simulink model "circleControlLoop"  (Simulink 7.5)
settings: Solver=ode1  StartTime=0.0  StopTime=15  FixedStep=0.001  RelTol=1e-3
PostLoadFcn:
  | , if any(exist('dsrtsu_mdlpostloadfcn', 'file') == [2, 3, 6]), try dsrtsu_mdlpostloadfcn('Execute', bdroot); catch fprintf('Error in PostLoadFcn (dsrtsu_mdlpostloadfcn) for model "%s":\n %s\n', bdroot, lasterr); end, end,
values from neighbouring files (symbols this model uses):
  kn = 1    [main.m]
  kt = 10    [main.m]
  r0 = Re-3.5    [main.m]
  Ts = 0.001    [main.m]
  Xr = [circXt.',circYt.',circXtd,circYtd,circXtdd,circYtdd]    [getCircle.m]
undefined symbols (not defined in the file or in its folder): DiscIntNeverNeededParam, xc, yc
libraries: rtilib1103 x12
settings Model: DSRTSU_INTERNAL_RTI_VER=360  DSRTSU_INTERNAL_RTI_TYPE=rti1103  Creator=daq  LastModifiedBy=daq  BufferReuse=off
settings OptimizationCC: BlockReduction=off  OptimizeBlockIOStorage=off  BufferReuse=off  ExpressionFolding=off  LocalBlockOutputs=off
settings HardwareCC: ProdIntDivRoundTo=Zero  ProdEndianess=BigEndian  ProdHWDeviceType=Generic->Custom  TargetIntDivRoundTo=Zero  TargetEndianess=BigEndian  TargetHWDeviceType=Generic->Custom
settings RTWCC: SystemTargetFile=rti1103.tlc  MakeCommand=make_rti  TemplateMakefile=rti1103.tmf  Description=dSPACE DS1103 Hardware Platform  ProcessScript=rti1103_make_rtw_hook
settings STFCustomTargetCC: ParMdlRefBuildCompliant=on  GeneratePreprocessorConditionals=Disable all  MatFileLogging=on  SystemTargetFile=rti1103.tlc
settings GRTTargetCC: CompOptLevelCompliant=off  ExtModeMexFile=noextcomm
settings CustomProperty: DataType=RTWOptions_EnumType_C__dSPACE_matlab_rti1103_tlc_rti1103_1InitialSimState  Value=RUN
settings EnumStrPairs: String=RUN

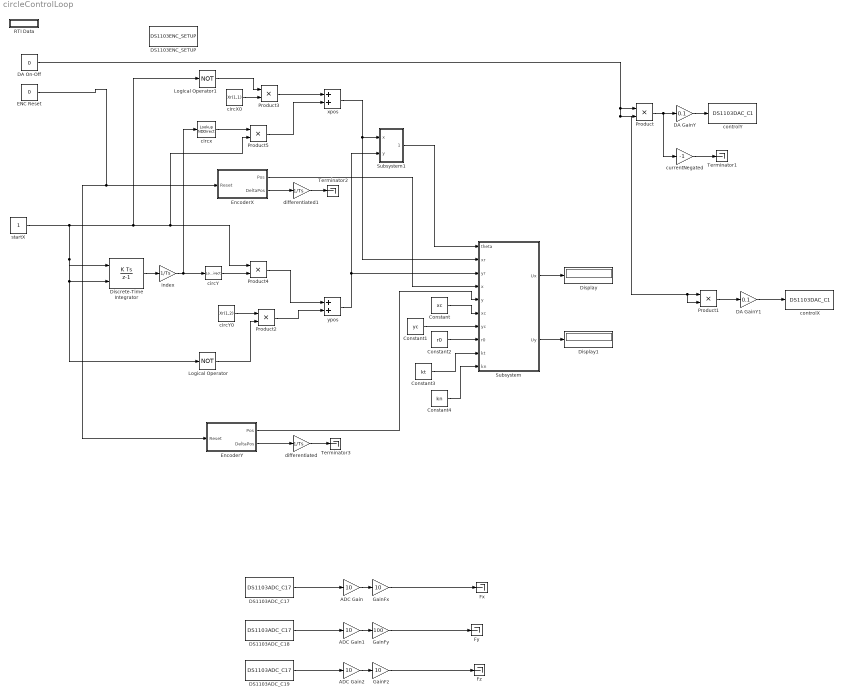
== system circleControlLoop ==
  " EncoderX" : Subsystem
  " EncoderY" : Subsystem
  ADC Gain : Gain  Gain=10  ParameterDataType=fixdt(1, 16)  ParameterScaling=2^0  OutDataType=fixdt(1, 16)  OutScaling=2^0
  ADC Gain1 : Gain  Gain=10  ParameterDataType=fixdt(1, 16)  ParameterScaling=2^0  OutDataType=fixdt(1, 16)  OutScaling=2^0
  ADC Gain2 : Gain  Gain=10  ParameterDataType=fixdt(1, 16)  ParameterScaling=2^0  OutDataType=fixdt(1, 16)  OutScaling=2^0
  Constant : Constant  Value=xc  OutDataType=fixdt(1, 16)  OutScaling=2^0
  Constant1 : Constant  Value=yc  OutDataType=fixdt(1, 16)  OutScaling=2^0
  Constant2 : Constant  Value=r0  OutDataType=fixdt(1, 16)  OutScaling=2^0
  Constant3 : Constant  Value=kt  OutDataType=fixdt(1, 16)  OutScaling=2^0
  Constant4 : Constant  Value=kn  OutDataType=fixdt(1, 16)  OutScaling=2^0
  DA GainY : Gain  Gain=0.1  ParameterDataType=fixdt(1, 16)  ParameterScaling=2^0  OutDataType=fixdt(1, 16)  OutScaling=2^0
  DA GainY1 : Gain  Gain=0.1  ParameterDataType=fixdt(1, 16)  ParameterScaling=2^0  OutDataType=fixdt(1, 16)  OutScaling=2^0
  DA On-Off : Constant  Value=0  OutDataType=fixdt(1, 16)  OutScaling=2^0
  DS1103ADC_C17 : rtilib1103/DS1103 MASTER PPC/DS1103ADC_C17  SystemSampleTime=-1  ChannelNo=17  TimerAPreTrigger=0  Reserved2=[]  Reserved3=[]  Reserved4=[]  DialogFcn=gui1103adc  UnitName={ 'DS1103ADC_C' }  UnitValues={ 17 }  DSProperties=struct('RTI',struct('Version',uint32(1),'BlockType',struct('isSLSource',uint8(1),'isSLSink',uint8(0),'isHWSource',uint8(1),'isHWSink',uint8(0),'isSetup',uint8(0),'isInline',uint8(1),'isNonInline',uint8(0),'isInterrupt',uint8(0),'isChannelwise',uint8(1)),'IOBoardType','DS1103MASTER','UnitType','ADC','Identifier','ADC','DialogType','ML','BlockSet','NONE','SlaveProcessor','NONE'))
  DS1103ADC_C18 : rtilib1103/DS1103 MASTER PPC/DS1103ADC_C17  SystemSampleTime=-1  ChannelNo=18  TimerAPreTrigger=0  Reserved2=[]  Reserved3=[]  Reserved4=[]  DialogFcn=gui1103adc  UnitName={ 'DS1103ADC_C' }  UnitValues={ 18 }  DSProperties=struct('RTI',struct('Version',uint32(1),'BlockType',struct('isSLSource',uint8(1),'isSLSink',uint8(0),'isHWSource',uint8(1),'isHWSink',uint8(0),'isSetup',uint8(0),'isInline',uint8(1),'isNonInline',uint8(0),'isInterrupt',uint8(0),'isChannelwise',uint8(1)),'IOBoardType','DS1103MASTER','UnitType','ADC','Identifier','ADC','DialogType','ML','BlockSet','NONE','SlaveProcessor','NONE'))
  DS1103ADC_C19 : rtilib1103/DS1103 MASTER PPC/DS1103ADC_C17  SystemSampleTime=-1  ChannelNo=19  TimerAPreTrigger=0  Reserved2=[]  Reserved3=[]  Reserved4=[]  DialogFcn=gui1103adc  UnitName={ 'DS1103ADC_C' }  UnitValues={ 19 }  DSProperties=struct('RTI',struct('Version',uint32(1),'BlockType',struct('isSLSource',uint8(1),'isSLSink',uint8(0),'isHWSource',uint8(1),'isHWSink',uint8(0),'isSetup',uint8(0),'isInline',uint8(1),'isNonInline',uint8(0),'isInterrupt',uint8(0),'isChannelwise',uint8(1)),'IOBoardType','DS1103MASTER','UnitType','ADC','Identifier','ADC','DialogType','ML','BlockSet','NONE','SlaveProcessor','NONE'))
  DS1103ENC_SETUP : rtilib1103/DS1103 MASTER PPC/DS1103ENC_SETUP  SystemSampleTime=-1  EncRange=0  Reserved1=[]  Reserved2=[]  Reserved3=[]  Reserved4=[]  DialogFcn=gui1103enc_setup  UnitName={ 'DS1103ENC_SETUP' }  UnitValues={ [] }  DSProperties=struct('RTI',struct('Version',uint32(1),'BlockType',struct('isSLSource',uint8(0),'isSLSink',uint8(0),'isHWSource',uint8(0),'isHWSink',uint8(0),'isSetup',uint8(0),'isInline',uint8(1),'isNonInline',uint8(0),'isInterrupt',uint8(0),'isChannelwise',uint8(0)),'IOBoardType','DS1103MASTER','UnitType','ENC','Identifier','ENCMASTER','DialogType','ML','BlockSet','NONE','SlaveProcessor','NONE'))
      settings: SignalType=[0 0 0 0 0 0 0]
  Discrete-Time Integrator : DiscreteIntegrator  ExternalReset=rising  SampleTime=Ts  OutDataType=fixdt(1, 16)  OutScaling=2^0  ICPrevOutput=DiscIntNeverNeededParam  ICPrevScaledInput=DiscIntNeverNeededParam
  Display : Display
  Display1 : Display
  ENC Reset : Constant  Value=0  OutDataType=fixdt(1, 16)  OutScaling=2^0
  Fx : Terminator
  Fy : Terminator
  Fz : Terminator
  GainFx : Gain  Gain=10  ParameterDataType=fixdt(1, 16)  ParameterScaling=2^0  OutDataType=fixdt(1, 16)  OutScaling=2^0
  GainFy : Gain  Gain=100  ParameterDataType=fixdt(1, 16)  ParameterScaling=2^0  OutDataType=fixdt(1, 16)  OutScaling=2^0
  GainFz : Gain  Gain=10  ParameterDataType=fixdt(1, 16)  ParameterScaling=2^0  OutDataType=fixdt(1, 16)  OutScaling=2^0
  Logical Operator : Logic  Operator=NOT  AllPortsSameDT=off  OutDataTypeMode=boolean  LogicDataType=fixdt(0, 8)  OutDataTypeStr=boolean
  Logical Operator1 : Logic  Operator=NOT  AllPortsSameDT=off  OutDataTypeMode=boolean  LogicDataType=fixdt(0, 8)  OutDataTypeStr=boolean
  Product{,1..5} (6 alike) : Product  OutDataType=fixdt(1, 16)  OutScaling=2^0  RndMeth=Zero
  RTI Data : Subsystem  Tag=struct('RTIDataServer',struct('RTIDataServerVs','2','RTIModelDescription','struct(''main'',''circleControlLoop'',''sub'',''circleControlLoop'',''isMp'',0)'))  LoadFcn="if exist('rtidc'), try,  rtidc('DataHostBlockClbLoad', gcbh); catch, disp(['Warning: ''LoadFcn'' for RTI Data block failed: ' lasterr]); end, end,"
      settings: CopyFcn="if exist('rtidc'), try,  rtidc('DataHostBlockClbCopy', gcbh); catch, disp(['Warning: ''CopyFcn'' for RTI Data block failed: ' lasterr]); end, end,"  DeleteFcn="if exist('rtidc'), try,  rtidc('DataHostBlockClbDelete', gcbh); catch, disp(['Warning: ''DeleteFcn'' for RTI Data block failed: ' lasterr]); end, end,"  ModelCloseFcn="if exist('rtidc'), try,  rtidc('DataHostBlockClbModelClose', gcbh); catch, disp(['Warning: ''ModelCloseFcn'' for RTI Data block failed: ' lasterr]); end, end,"  PreSaveFcn="if exist('rtidc'), try,  rtidc('DataHostBlockClbPreSave', gcbh); catch, disp(['Warning: ''PreSaveFcn'' for RTI Data block failed: ' lasterr]); end, end,"  PostSaveFcn="if exist('rtidc'), try,  rtidc('DataHostBlockClbPostSave', gcbh); catch, disp(['Warning: ''PostSaveFcn'' for RTI Data block failed: ' lasterr]); end, end,"  NameChangeFcn="if exist('rtidc'), try,  rtidc('DataHostBlockClbNameChange', gcbh); catch, disp(['Warning: ''NameChangeFcn'' for RTI Data block failed: ' lasterr]); end, end,"
      mask Type: RTI_DATA_HOST
      mask Description:
      | RTI Data Block.
      | This block is used by RTI to store internal model-dependent data.
      | Please keep this block on the root level of the model. Deleting this block will result in data loss.
      | 
      | NEVER DELETE OR COPY THIS BLOCK!
      mask Help:
      | RTI Data Block.
      | This block is used by RTI to store internal model-dependent data.
      | Please keep this block on the root level of the model. Deleting this block will result in data loss.
      | 
      | NEVER DELETE OR COPY THIS BLOCK!
      mask Display:
      | text(0.5, 0.5, 'RTI Data', 'HorizontalAlignment', 'center');
      | plot([1 0]);
  Subsystem : Subsystem
  Subsystem1 : Subsystem
  Terminator1 : Terminator
  Terminator2 : Terminator
  Terminator3 : Terminator
  circX0 : Constant  Value=Xr(1,1)  OutDataType=fixdt(1, 16)  OutScaling=2^0
  circY : LookupNDDirect  NumberOfTableDimensions=1  Table=Xr(:,2)
  circY0 : Constant  Value=Xr(1,2)  OutDataType=fixdt(1, 16)  OutScaling=2^0
  circx : LookupNDDirect  NumberOfTableDimensions=1  Table=Xr(:,1)
  controlX : rtilib1103/DS1103 MASTER PPC/DS1103DAC_C1  SystemSampleTime=-1  ChannelNo=1  InitValue=0  TermMode=0  TermValue=0  Reserved1=[]  Reserved2=[]  Reserved3=[]  Reserved4=[]  DialogFcn=gui1103dac  UnitName={ 'DS1103DAC_C' }  UnitValues={ 1 }  DSProperties=struct('RTI',struct('Version',uint32(1),'BlockType',struct('isSLSource',uint8(0),'isSLSink',uint8(1),'isHWSource',uint8(0),'isHWSink',uint8(1),'isSetup',uint8(0),'isInline',uint8(1),'isNonInline',uint8(0),'isInterrupt',uint8(0),'isChannelwise',uint8(1)),'IOBoardType','DS1103MASTER','UnitType','DAC','Identifier','DAC','DialogType','ML','BlockSet','NONE','SlaveProcessor','NONE'))
  controlY : rtilib1103/DS1103 MASTER PPC/DS1103DAC_C1  SystemSampleTime=-1  ChannelNo=2  InitValue=0  TermMode=1  TermValue=0  Reserved1=[]  Reserved2=[]  Reserved3=[]  Reserved4=[]  DialogFcn=gui1103dac  UnitName={ 'DS1103DAC_C' }  UnitValues={ 2 }  DSProperties=struct('RTI',struct('Version',uint32(1),'BlockType',struct('isSLSource',uint8(0),'isSLSink',uint8(1),'isHWSource',uint8(0),'isHWSink',uint8(1),'isSetup',uint8(0),'isInline',uint8(1),'isNonInline',uint8(0),'isInterrupt',uint8(0),'isChannelwise',uint8(1)),'IOBoardType','DS1103MASTER','UnitType','DAC','Identifier','DAC','DialogType','ML','BlockSet','NONE','SlaveProcessor','NONE'))
  currentNegated : Gain  Gain=-1  ParameterDataType=fixdt(1, 16)  ParameterScaling=2^0  OutDataType=fixdt(1, 16)  OutScaling=2^0
  differentiated : Gain  Gain=1/Ts  ParameterDataType=fixdt(1, 16)  ParameterScaling=2^0  OutDataType=fixdt(1, 16)  OutScaling=2^0
  differentiated1 : Gain  Gain=1/Ts  ParameterDataType=fixdt(1, 16)  ParameterScaling=2^0  OutDataType=fixdt(1, 16)  OutScaling=2^0
  index : Gain  Gain=1/Ts  ParameterDataType=fixdt(1, 16)  ParameterScaling=2^0  OutDataType=fixdt(1, 16)  OutScaling=2^0
  startX : Constant  OutDataType=fixdt(1, 16)  OutScaling=2^0
  xpos : Sum  OutDataType=fixdt(1, 16)  OutScaling=2^-10
  ypos : Sum  OutDataType=fixdt(1, 16)  OutScaling=2^-10
  wires:
  DA GainY/1 -> controlY/1
  Product/1 -> DA GainY/1, currentNegated/1
  DA On-Off/1 -> Product/1, Product/2, Product1/1, Product1/2
  ENC Reset/1 -> " EncoderX"/1(Reset), " EncoderY"/1(Reset)
  DS1103ADC_C18/1 -> ADC Gain1/1
  GainFz/1 -> Fz/1
  DS1103ADC_C17/1 -> ADC Gain/1
  ADC Gain/1 -> GainFx/1
  ADC Gain1/1 -> GainFy/1
  ADC Gain2/1 -> GainFz/1
  GainFy/1 -> Fy/1
  currentNegated/1 -> Terminator1/1
  " EncoderY"/2(DeltaPos) -> differentiated/1
  GainFx/1 -> Fx/1
  DS1103ADC_C19/1 -> ADC Gain2/1
  startX/1 -> Discrete-Time Integrator/1, Discrete-Time Integrator/2, Logical Operator/1, Logical Operator1/1, Product4/1, Product5/2
  Discrete-Time Integrator/1 -> index/1
  index/1 -> circY/1, circx/1
  differentiated1/1 -> Terminator2/1
  differentiated/1 -> Terminator3/1
  Product1/1 -> DA GainY1/1
  DA GainY1/1 -> controlX/1
  circY0/1 -> Product2/1
  Product2/1 -> ypos/2
  Logical Operator/1 -> Product2/2
  circX0/1 -> Product3/2
  Product3/1 -> xpos/1
  Logical Operator1/1 -> Product3/1
  circY/1 -> Product4/2
  Product4/1 -> ypos/1
  circx/1 -> Product5/1
  Product5/1 -> xpos/2
  " EncoderX"/2(DeltaPos) -> differentiated1/1
  xpos/1 -> Subsystem/2(xr), Subsystem1/1(x)
  ypos/1 -> Subsystem1/2(y), Subsystem/3(yr)
  Subsystem1/1(Out1) -> Subsystem/1(theta)
  " EncoderX"/1(Pos) -> Subsystem/4(x)
  " EncoderY"/1(Pos) -> Subsystem/5(y)
  Constant/1 -> Subsystem/6(xc)
  Constant1/1 -> Subsystem/7(yc)
  Constant2/1 -> Subsystem/8(r0)
  Constant3/1 -> Subsystem/9(kt)
  Constant4/1 -> Subsystem/10(kn)
  Subsystem/1(Ux) -> Display/1
  Subsystem/2(Uy) -> Display1/1

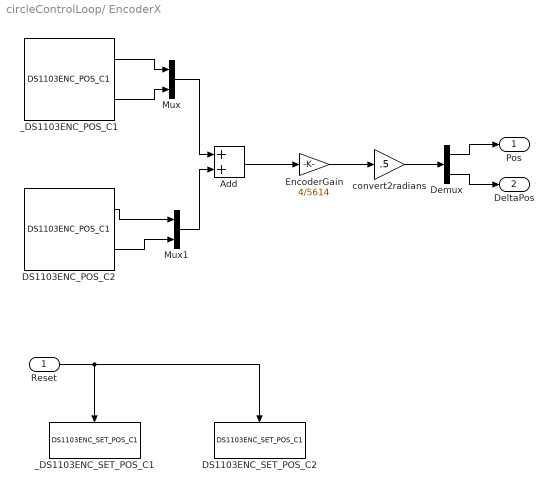
== system circleControlLoop/ EncoderX ==
  Reset : Inport
  Add : Sum  OutDataType=fixdt(1, 16)  OutScaling=2^-10
  DS1103ENC_POS_C2 : rtilib1103/DS1103 MASTER PPC/DS1103ENC_POS_C1  SystemSampleTime=-1  ChannelNo=2  PosValue=0  Reserved1=[]  Reserved2=[]  Reserved3=[]  Reserved4=[]  DialogFcn=gui1103enc_pos  UnitName={ 'DS1103ENC_POS_C' }  UnitValues={ 2 }  DSProperties=struct('RTI',struct('Version',uint32(1),'BlockType',struct('isSLSource',uint8(1),'isSLSink',uint8(0),'isHWSource',uint8(1),'isHWSink',uint8(0),'isSetup',uint8(0),'isInline',uint8(1),'isNonInline',uint8(0),'isInterrupt',uint8(0),'isChannelwise',uint8(1)),'IOBoardType','DS1103MASTER','UnitType','ENC','Identifier','ENCPOSCH','DialogType','ML','BlockSet','NONE','SlaveProcessor','NONE'))
  DS1103ENC_SET_POS_C2 : rtilib1103/DS1103 MASTER PPC/DS1103ENC_SET_POS_C1  SystemSampleTime=-1  ChannelNo=2  PosValue=0  Reserved1=[]  Reserved2=[]  Reserved3=[]  Reserved4=[]  DialogFcn=gui1103enc_set_pos  UnitName={ 'DS1103ENC_SET_POS_C' }  UnitValues={ 2 }  DSProperties=struct('RTI',struct('Version',uint32(1),'BlockType',struct('isSLSource',uint8(0),'isSLSink',uint8(1),'isHWSource',uint8(0),'isHWSink',uint8(1),'isSetup',uint8(0),'isInline',uint8(1),'isNonInline',uint8(0),'isInterrupt',uint8(0),'isChannelwise',uint8(1)),'IOBoardType','DS1103MASTER','UnitType','ENC','Identifier','ENCRESET','DialogType','ML','BlockSet','NONE','SlaveProcessor','NONE'))
  Demux : Demux  Outputs=2
  EncoderGain : Gain  Gain=4/5614  SaturateOnIntegerOverflow=on  OutDataTypeStr=Inherit: Same as input  ParamDataTypeStr=Inherit: Same as input
  Mux : Mux  Inputs=2
  Mux1 : Mux  Inputs=2
  _DS1103ENC_POS_C1 : rtilib1103/DS1103 MASTER PPC/DS1103ENC_POS_C1  SystemSampleTime=-1  ChannelNo=1  PosValue=0  Reserved1=[]  Reserved2=[]  Reserved3=[]  Reserved4=[]  DialogFcn=gui1103enc_pos  UnitName={ 'DS1103ENC_POS_C' }  UnitValues={ 1 }  DSProperties=struct('RTI',struct('Version',uint32(1),'BlockType',struct('isSLSource',uint8(1),'isSLSink',uint8(0),'isHWSource',uint8(1),'isHWSink',uint8(0),'isSetup',uint8(0),'isInline',uint8(1),'isNonInline',uint8(0),'isInterrupt',uint8(0),'isChannelwise',uint8(1)),'IOBoardType','DS1103MASTER','UnitType','ENC','Identifier','ENCPOSCH','DialogType','ML','BlockSet','NONE','SlaveProcessor','NONE'))
  _DS1103ENC_SET_POS_C1 : rtilib1103/DS1103 MASTER PPC/DS1103ENC_SET_POS_C1  SystemSampleTime=-1  ChannelNo=1  PosValue=0  Reserved1=[]  Reserved2=[]  Reserved3=[]  Reserved4=[]  DialogFcn=gui1103enc_set_pos  UnitName={ 'DS1103ENC_SET_POS_C' }  UnitValues={ 1 }  DSProperties=struct('RTI',struct('Version',uint32(1),'BlockType',struct('isSLSource',uint8(0),'isSLSink',uint8(1),'isHWSource',uint8(0),'isHWSink',uint8(1),'isSetup',uint8(0),'isInline',uint8(1),'isNonInline',uint8(0),'isInterrupt',uint8(0),'isChannelwise',uint8(1)),'IOBoardType','DS1103MASTER','UnitType','ENC','Identifier','ENCRESET','DialogType','ML','BlockSet','NONE','SlaveProcessor','NONE'))
  "convert2radians " : Gain  Gain=.5
  Pos : Outport
  DeltaPos : Outport  Port=2
  wires:
  _DS1103ENC_POS_C1/1 -> Mux/1
  _DS1103ENC_POS_C1/2 -> Mux/2
  EncoderGain/1 -> "convert2radians "/1
  "convert2radians "/1 -> Demux/1
  Reset/1 -> _DS1103ENC_SET_POS_C1/Trigger, DS1103ENC_SET_POS_C2/Trigger
  Mux/1 -> Add/1
  Demux/1 -> Pos/1
  Demux/2 -> DeltaPos/1
  Mux1/1 -> Add/2
  DS1103ENC_POS_C2/1 -> Mux1/1
  DS1103ENC_POS_C2/2 -> Mux1/2
  Add/1 -> EncoderGain/1

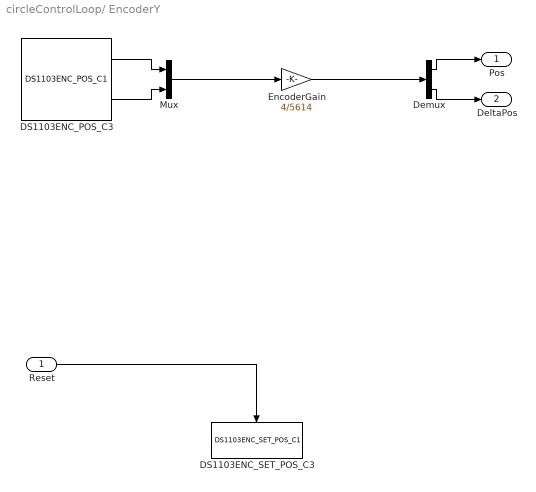
== system circleControlLoop/ EncoderY ==
  Reset : Inport
  DS1103ENC_POS_C3 : rtilib1103/DS1103 MASTER PPC/DS1103ENC_POS_C1  SystemSampleTime=-1  ChannelNo=3  PosValue=0  Reserved1=[]  Reserved2=[]  Reserved3=[]  Reserved4=[]  DialogFcn=gui1103enc_pos  UnitName={ 'DS1103ENC_POS_C' }  UnitValues={ 3 }  DSProperties=struct('RTI',struct('Version',uint32(1),'BlockType',struct('isSLSource',uint8(1),'isSLSink',uint8(0),'isHWSource',uint8(1),'isHWSink',uint8(0),'isSetup',uint8(0),'isInline',uint8(1),'isNonInline',uint8(0),'isInterrupt',uint8(0),'isChannelwise',uint8(1)),'IOBoardType','DS1103MASTER','UnitType','ENC','Identifier','ENCPOSCH','DialogType','ML','BlockSet','NONE','SlaveProcessor','NONE'))
  DS1103ENC_SET_POS_C3 : rtilib1103/DS1103 MASTER PPC/DS1103ENC_SET_POS_C1  SystemSampleTime=-1  ChannelNo=3  PosValue=0  Reserved1=[]  Reserved2=[]  Reserved3=[]  Reserved4=[]  DialogFcn=gui1103enc_set_pos  UnitName={ 'DS1103ENC_SET_POS_C' }  UnitValues={ 3 }  DSProperties=struct('RTI',struct('Version',uint32(1),'BlockType',struct('isSLSource',uint8(0),'isSLSink',uint8(1),'isHWSource',uint8(0),'isHWSink',uint8(1),'isSetup',uint8(0),'isInline',uint8(1),'isNonInline',uint8(0),'isInterrupt',uint8(0),'isChannelwise',uint8(1)),'IOBoardType','DS1103MASTER','UnitType','ENC','Identifier','ENCRESET','DialogType','ML','BlockSet','NONE','SlaveProcessor','NONE'))
  Demux : Demux  Outputs=2
  EncoderGain : Gain  Gain=4/5614  SaturateOnIntegerOverflow=on  OutDataTypeStr=Inherit: Same as input  ParamDataTypeStr=Inherit: Same as input
  Mux : Mux  Inputs=2
  Pos : Outport
  DeltaPos : Outport  Port=2
  wires:
  Mux/1 -> EncoderGain/1
  Demux/2 -> DeltaPos/1
  Demux/1 -> Pos/1
  Reset/1 -> DS1103ENC_SET_POS_C3/Trigger
  EncoderGain/1 -> Demux/1
  DS1103ENC_POS_C3/2 -> Mux/2
  DS1103ENC_POS_C3/1 -> Mux/1

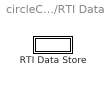
== system circleControlLoop/RTI Data ==
  RTI Data Store : Subsystem  Tag="struct('private',struct('version',struct('dsVer',uint32(2),'dsVerCreation',uint32(2),'RTI',struct('ver','6.5','type','RTI1103')),'access',struct('type','Model','isPerm',1,'created',['16-Oct-2016 18:11:40'],'modified',['13-Feb-2017 22:44:32'],'location','')),'public',struct('main',struct('data',[]),'sub',struct('name',{{'circleControlLoop'}},'data',{{struct('TH',struct('thTaskInfo',struct('taskType',{'TIMER','HWINT','TMRINT','SWINT'},'tasksNumOf',{1,0,0,0},'srcIds',{{'TIMERA'},{},{},{}},'taskNames',{{['Timer Task 1']},{},{},{}})),'th_tc',struct('dataType','TASK','taskGroupId','','taskGroupList',{{}},'taskSchedulingPolicy','FCFS','taskType','TIMER','blkh',-1,'srcId','TIMERA','srcSgnName',['Timer A interrupt'],'srcCpuName','','taskName',['Timer Task 1  [0.01] s'],'taskNameDisplayExt','','smplTime',0.01,'smplTimeOffs',0,'hasFixedPriority',0,'priority',1,'hasFixedOvc',0,'ovcType',1,'ovcMax',1),'tc_th',struct('dataType','TASK','taskGroupId','','taskGroupList',{{}},'taskSchedulingPolicy','FCFS','taskType','TIMER','blkh',-1,'srcId','TIMERA','srcSgnName',['Timer A interrupt'],'srcCpuName','','taskName',['Timer Task 1  [0.01] s'],'taskNameDisplayExt','','smplTime',0.01,'smplTimeOffs',0,'hasFixedPriority',0,'priority',1,'hasFixedOvc',0,'ovcType',1,'ovcMax',1))}})))"
      mask Type: RTI_DATA_STORE
      mask Description:
      | RTI Data Store Block. This block is used by RTI to store internal model dependent data. Deleting this block will result in data loss.
      | 
      | NEVER DELETE, COPY, OR MODIFY THIS BLOCK!
      mask Help:
      | RTI Data Store Block. This block is used by RTI to store internal model dependent data. Deleting this block will result in data loss.
      | 
      | NEVER DELETE, COPY, OR MODIFY THIS BLOCK!
      mask Display: text(0.5, 0.5, ' ', 'HorizontalAlignment', 'center');

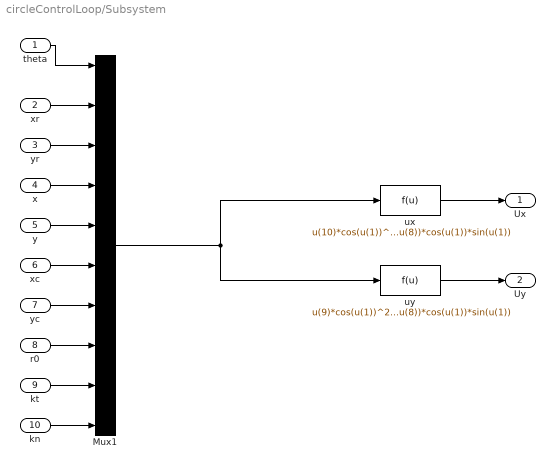
== system circleControlLoop/Subsystem ==
  theta : Inport
  xr : Inport  Port=2
  yr : Inport  Port=3
  x : Inport  Port=4
  y : Inport  Port=5
  xc : Inport  Port=6
  yc : Inport  Port=7
  r0 : Inport  Port=8
  kt : Inport  Port=9
  kn : Inport  Port=10
  Mux1 : Mux  Inputs=10
  ux : Fcn  Expr=u(10)*cos(u(1))^2*conj(u(6)) - u(10)*cos(u(1))^2*conj(u(4)) + u(10)*cos(u(1))^2*conj(u(5)) - u(10)*cos(u(1))^2*conj(u(3)) - u(9)*conj(u(4))*sin(u(1))^2 + u(9)*conj(u(2))*sin(u(1))^2 + u(10)*cos(conj(u(1)))*conj(u(8))*cos(u(1))^2 - u(10)*cos(u(1))*conj(u(4))*sin(u(1)) + u(10)*cos(u(1))*conj(u(2))*sin(u(1)) - u(10)*cos(u(1))*conj(u(5))*sin(u(1)) + u(9)*cos(u(1))*conj(u(5))*sin(u(1)) + u(10)*cos(u(1))*conj(u(7))*sin(u(1)) - u(9)*cos(u(1))*conj(u(3))*sin(u(1)) + u(10)*sin(conj(u(1)))*conj(u(8))*cos(u(1))*sin(u(1))
  uy : Fcn  Expr=u(9)*cos(u(1))^2*conj(u(3)) - u(9)*cos(u(1))^2*conj(u(5)) - u(10)*conj(u(4))*sin(u(1))^2 + u(10)*conj(u(2))*sin(u(1))^2 - u(10)*conj(u(5))*sin(u(1))^2 + u(10)*conj(u(7))*sin(u(1))^2 + u(10)*sin(conj(u(1)))*conj(u(8))*sin(u(1))^2 - u(10)*cos(u(1))*conj(u(4))*sin(u(1)) + u(9)*cos(u(1))*conj(u(4))*sin(u(1)) + u(10)*cos(u(1))*conj(u(6))*sin(u(1)) - u(9)*cos(u(1))*conj(u(2))*sin(u(1)) + u(10)*cos(u(1))*conj(u(5))*sin(u(1)) - u(10)*cos(u(1))*conj(u(3))*sin(u(1)) + u(10)*cos(conj(u(1)))*conj(u(8))*cos(u(1))*sin(u(1))
  Ux : Outport  OutDataType=fixdt(1, 16)  OutScaling=2^0
  Uy : Outport  Port=2  OutDataType=fixdt(1, 16)  OutScaling=2^0
  wires:
  xr/1 -> Mux1/2
  yr/1 -> Mux1/3
  theta/1 -> Mux1/1
  x/1 -> Mux1/4
  y/1 -> Mux1/5
  xc/1 -> Mux1/6
  yc/1 -> Mux1/7
  r0/1 -> Mux1/8
  kt/1 -> Mux1/9
  kn/1 -> Mux1/10
  Mux1/1 -> uy/1, ux/1
  ux/1 -> Ux/1
  uy/1 -> Uy/1

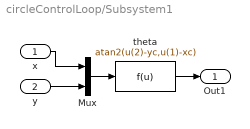
== system circleControlLoop/Subsystem1 ==
  x : Inport
  y : Inport  Port=2
  Mux : Mux  Inputs=2
  theta : Fcn  Expr=atan2(u(2)-yc,u(1)-xc)
  Out1 : Outport
  wires:
  Mux/1 -> theta/1
  x/1 -> Mux/1
  y/1 -> Mux/2
  theta/1 -> Out1/1

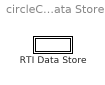
== system circleControlLoop/RTI Data/RTI Data Store ==
  RTI Data Store : Subsystem
      mask Type: RTI_DATA_STORE
      mask Description:
      | RTI Data Store Block. This block is used by RTI to store internal model dependent data. Deleting this block will result in data loss.
      | 
      | NEVER DELETE, COPY, OR MODIFY THIS BLOCK!
      mask Help:
      | RTI Data Store Block. This block is used by RTI to store internal model dependent data. Deleting this block will result in data loss.
      | 
      | NEVER DELETE, COPY, OR MODIFY THIS BLOCK!
      mask Display: text(0.5, 0.5, ' ', 'HorizontalAlignment', 'center');

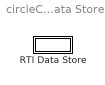
== system circleControlLoop/RTI Data/RTI Data Store/RTI Data Store ==
  RTI Data Store : Subsystem
      mask Type: RTI_DATA_STORE
      mask Description:
      | RTI Data Store Block. This block is used by RTI to store internal model dependent data. Deleting this block will result in data loss.
      | 
      | NEVER DELETE, COPY, OR MODIFY THIS BLOCK!
      mask Help:
      | RTI Data Store Block. This block is used by RTI to store internal model dependent data. Deleting this block will result in data loss.
      | 
      | NEVER DELETE, COPY, OR MODIFY THIS BLOCK!
      mask Display: text(0.5, 0.5, ' ', 'HorizontalAlignment', 'center');

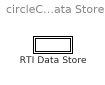
== system circleControlLoop/RTI Data/RTI Data Store/RTI Data Store/RTI Data Store ==
  RTI Data Store : Subsystem
      mask Type: RTI_DATA_STORE
      mask Description:
      | RTI Data Store Block. This block is used by RTI to store internal model dependent data. Deleting this block will result in data loss.
      | 
      | NEVER DELETE, COPY, OR MODIFY THIS BLOCK!
      mask Help:
      | RTI Data Store Block. This block is used by RTI to store internal model dependent data. Deleting this block will result in data loss.
      | 
      | NEVER DELETE, COPY, OR MODIFY THIS BLOCK!
      mask Display: text(0.5, 0.5, ' ', 'HorizontalAlignment', 'center');

== system circleControlLoop/RTI Data/RTI Data Store/RTI Data Store/RTI Data Store/RTI Data Store ==
